simulink model "ipLink2"  (Simulink 7.4)
settings: Solver=FixedStepDiscrete  StartTime=0.0  StopTime=inf  FixedStep=1  RelTol=1e-3
settings Model: Creator=tyler  LastModifiedBy=tyler
settings RTWCC: SystemTargetFile=nrt.tlc  TemplateMakefile=nrt_unix.tmf  Description=Nokia Real-Time Target  ProcessScript=nrt_make_rtw_hook
settings STFCustomTargetCC: ModelReferenceCompliant=off  GeneratePreprocessorConditionals=Disable all  MatFileLogging=on  SystemTargetFile=nrt.tlc
settings GRTTargetCC: ModelReferenceCompliant=off  ParMdlRefBuildCompliant=off  CompOptLevelCompliant=off
settings CustomProperty: DataType=string  Value=-lm -ldl
settings EnumStrPairs: String=PC

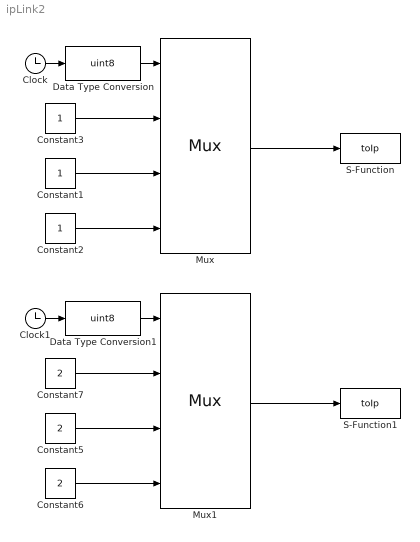
== system ipLink2 ==
  Clock : Clock
      settings: Decimation=10
  Clock1 : Clock
      settings: Decimation=10
  Constant1 : Constant  OutDataTypeMode=uint8  OutDataType=fixdt(1, 16)  OutScaling=2^0  OutDataTypeStr=uint8
  Constant2 : Constant  OutDataTypeMode=uint8  OutDataType=fixdt(1, 16)  OutScaling=2^0  OutDataTypeStr=uint8
  Constant3 : Constant  OutDataTypeMode=uint8  OutDataType=fixdt(1, 16)  OutScaling=2^0  OutDataTypeStr=uint8
  Constant5 : Constant  Value=2  OutDataTypeMode=uint8  OutDataType=fixdt(1, 16)  OutScaling=2^0  OutDataTypeStr=uint8
  Constant6 : Constant  Value=2  OutDataTypeMode=uint8  OutDataType=fixdt(1, 16)  OutScaling=2^0  OutDataTypeStr=uint8
  Constant7 : Constant  Value=2  OutDataTypeMode=uint8  OutDataType=fixdt(1, 16)  OutScaling=2^0  OutDataTypeStr=uint8
  Data Type Conversion : DataTypeConversion  OutDataTypeMode=uint8  OutDataType=fixdt(1, 16)  OutScaling=2^0  OutDataTypeStr=uint8
  Data Type Conversion1 : DataTypeConversion  OutDataTypeMode=uint8  OutDataType=fixdt(1, 16)  OutScaling=2^0  OutDataTypeStr=uint8
  Mux : Mux
  Mux1 : Mux
  S-Function : S-Function  FunctionName=toIp  Parameters='127.0.0.1','6665'  EnableBusSupport=off
  S-Function1 : S-Function  FunctionName=toIp  Parameters='127.0.0.1','6666'  EnableBusSupport=off
  wires:
  Mux/1 -> S-Function/1
  Constant1/1 -> Mux/3
  Constant2/1 -> Mux/4
  Constant3/1 -> Mux/2
  Mux1/1 -> S-Function1/1
  Constant5/1 -> Mux1/3
  Constant6/1 -> Mux1/4
  Constant7/1 -> Mux1/2
  Clock/1 -> Data Type Conversion/1
  Data Type Conversion/1 -> Mux/1
  Clock1/1 -> Data Type Conversion1/1
  Data Type Conversion1/1 -> Mux1/1
